simulink model "simulationQ8"  (R2023a)
settings: Solver=ode45  StartTime=0.0  StopTime=10.0  RelTol=1e-3  EnableMultiTasking=on
values from neighbouring files (symbols this model uses):
  A = [0 0 0 0 0 1 -0.0174048595758 0 -0.0173759205618 -232.025201375 0 20.7861247087 ... (25 elements, 5x5)]    [fp_lin_matrices_fit3.mat]
  A_controler = A-B*K-L*C    [Main.m]    (also in Question9_Experiments.m; simulater.m)
  B = [0 0 0 0 333.33674813]    [fp_lin_matrices_fit3.mat]
  B_controler = L    [Main.m]    (also in Question9_Experiments.m; simulater.m)
  C = eye(5)    [Main.m]    (also in Question9_Experiments.m; fp_lin_matrices_fit3.mat = [1  0  0  0  0; 0  0  1  0  0]; simulater.m)
  C_controler = -K    [Main.m]    (also in Question9_Experiments.m; simulater.m)
  D = [0 0 0 0 0]'    [Main.m]    (also in Question9_Experiments.m; fp_lin_matrices_fit3.mat = [0 0]; simulater.m)
  D_controler = zeros(1,5)    [Main.m]    (also in Question9_Experiments.m; simulater.m)
  x0 = [0.1 0 0 0 0]'    [Main.m]    (also in Question9_Experiments.m; simulater.m)
settings Model: Creator=Alunos  LastModifiedBy=joaodias
settings SolverCC: AlgebraicLoopSolver=TrustRegion
settings DataIOCC: LimitDataPoints=on  SaveFormat=Array  ReturnWorkspaceOutputs=off
settings OptimizationCC: LifeSpan=inf
settings DebuggingCC: UnconnectedInputMsg=warning  UnconnectedOutputMsg=warning  UnconnectedLineMsg=warning  SFUnexpectedBacktrackingDiag=warning  SFNoUnconditionalDefaultTransitionDiag=warning  SFExecutionAtInitializationDiag=none  ArithmeticOperatorsInVariantConditions=warning
settings HardwareCC: ProdBitPerPointer=32  ProdBitPerSizeT=32  ProdBitPerPtrDiffT=32  ProdLargestAtomicFloat=None  ProdIntDivRoundTo=Undefined  ProdEndianess=Unspecified  ProdWordSize=32  ProdHWDeviceType=32-bit Generic
settings ModelReferenceCC: PropagateSignalLabelsOutOfModel=off
settings SFSimCC: SimUseLocalCustomCode=off  CustomCodeUndefinedFunction=UseInterfaceOnly
settings RTWCC: RTWUseLocalCustomCode=off
settings CodeAppCC: StateflowObjectComments=on
settings GRTTargetCC: TargetLangStandard=C89/C90 (ANSI)
settings ConfigComp: CovMetricSettings=dw  CovSaveCumulativeToWorkspaceVar=on  CovSaveSingleToWorkspaceVar=on  CovExternalEMLEnable=off

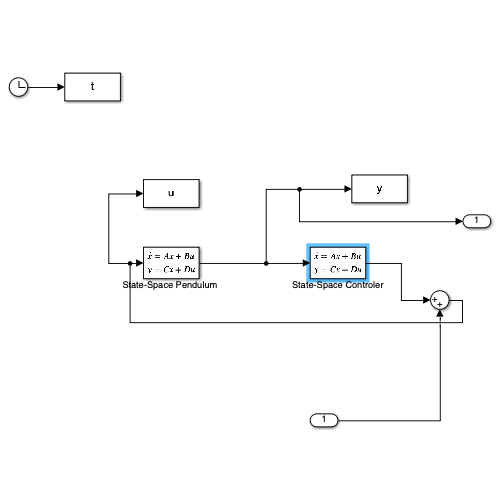
[thumbnail: Simulink's stored preview of the top-level diagram]
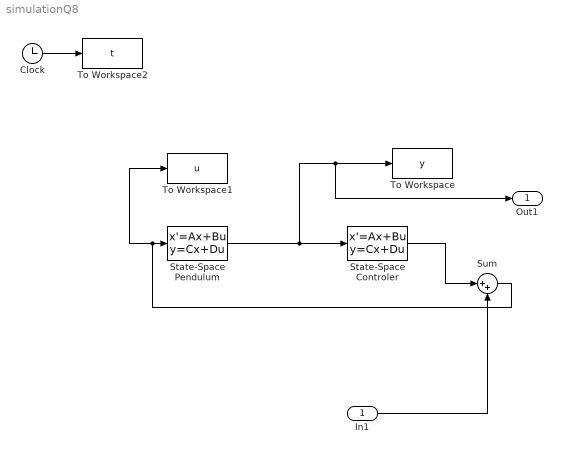
== system simulationQ8 ==
  In1 : Inport
  Clock : Clock
  "State-Space Controler " : StateSpace  A=A_controler  B=B_controler  C=C_controler  D=D_controler  InitialCondition=0
  "State-Space Pendulum " : StateSpace  A=A  B=B  C=C  D=D  InitialCondition=x0
  Sum : Sum  Inputs=|++
  To Workspace : ToWorkspace  VariableName=y  SampleTime=-1
  To Workspace1 : ToWorkspace  VariableName=u  SampleTime=-1
  To Workspace2 : ToWorkspace  VariableName=t  SampleTime=-1
  Out1 : Outport
  wires:
  "State-Space Pendulum "/1 -> "State-Space Controler "/1, Out1/1, To Workspace/1
  Clock/1 -> To Workspace2/1
  In1/1 -> Sum/2
  "State-Space Controler "/1 -> Sum/1
  Sum/1 -> To Workspace1/1, "State-Space Pendulum "/1
